simulink model "LabB_CheckCommunications"  (R2018b)
settings: Solver=FixedStepDiscrete  StartTime=0.0  StopTime=Inf  FixedStep=fSamplingPeriod  RelTol=1e-3  EnableMultiTasking=on
values from neighbouring files (symbols this model uses):
  fSamplingPeriod = 0.005    [LabB_ObserverOverSimulator_Discrete_Parameters.m]    (also in LabB_PIDOverRobot_Parameters.m)
undefined symbols (not defined in the file or in its folder): DiscIntNeverNeededParam
libraries: simulink_extras x3, MinSegLibrary_M2V3 x3
settings Model: SimulationMode=external  ExtModeTrigDuration=2  Creator=Alec  LastModifiedBy=pyry
settings DataIOCC: LimitDataPoints=on  SaveFormat=Array
settings OptimizationCC: PassReuseOutputArgsAs=Individual arguments  ExpressionDepthLimit=2147483647  MaxStackSize=64
settings DebuggingCC: UnderspecifiedInitializationDetection=Classic  MergeDetectMultiDrivingBlocksExec=none  ParameterTunabilityLossMsg=error  StateNameClashWarn=warning  SFUnexpectedBacktrackingDiag=warning  SFNoUnconditionalDefaultTransitionDiag=warning  SFExecutionAtInitializationDiag=none
settings HardwareCC: ProdBitPerInt=16  ProdBitPerPointer=16  ProdBitPerSizeT=16  ProdBitPerPtrDiffT=16  ProdLargestAtomicFloat=None  ProdWordSize=8  ProdHWDeviceType=Atmel->AVR
settings ModelReferenceCC: PropagateSignalLabelsOutOfModel=off
settings SFSimCC: SimUseLocalCustomCode=off  MATLABDynamicMemAlloc=off
settings RTWCC: SystemTargetFile=ert.tlc  HardwareBoard=Arduino Mega 2560  TemplateMakefile=ert_default_tmf  GenerateReport=on  RTWVerbose=off  RTWUseLocalCustomCode=off  Toolchain=Arduino AVR  BuildConfiguration=Faster Runs  IncludeHyperlinkInReport=on  LaunchReport=on  GenerateTraceInfo=on  GenerateTraceReport=on  GenerateTraceReportSl=on  GenerateTraceReportSf=on  GenerateTraceReportEml=on
settings CodeAppCC: ForceParamTrailComments=on  IgnoreCustomStorageClasses=off  OperatorAnnotations=on  SimulinkDataObjDesc=on  SFDataObjDesc=on  MATLABFcnDesc=on  CustomSymbolStrType=$N$R$M  InsertBlockDesc=on  StateflowObjectComments=on  MATLABSourceComments=on  InternalIdentifier=Classic
settings ERTTargetCC: SupportContinuousTime=on  SupportVariableSizeSignals=on
settings ConfigComp: CovMetricSettings=dw  CovHtmlReporting=on  CovSaveCumulativeToWorkspaceVar=on  CovSaveSingleToWorkspaceVar=on  CovExternalEMLEnable=off

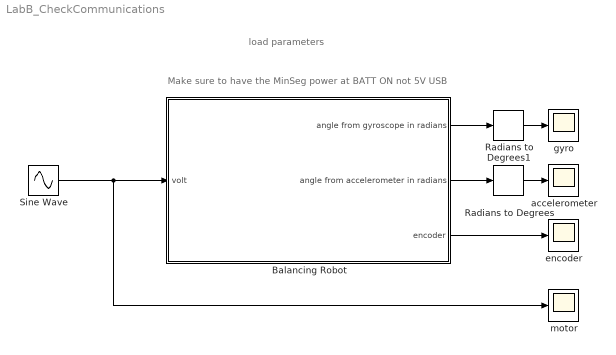
== system LabB_CheckCommunications ==
  note: Make sure to have the MinSeg power at BATT ON not 5V USB
  note: load parameters
  Balancing Robot : Subsystem
  Radians to Degrees : simulink_extras/Transformations/Radians to Degrees
  Radians to Degrees1 : simulink_extras/Transformations/Radians to Degrees
  Sine Wave : Sin  Amplitude=2  Frequency=pi/3  SampleTime=fSamplingPeriod
  accelerometer : Scope
  encoder : Scope
  gyro : Scope
  motor : Scope
  wires:
  Balancing Robot/1(angle from gyroscope in radians) -> Radians to Degrees1/1
  Balancing Robot/2(angle from accelerometer in radians) -> Radians to Degrees/1
  Balancing Robot/3(encoder) -> encoder/1
  Radians to Degrees1/1 -> gyro/1
  Radians to Degrees/1 -> accelerometer/1
  Sine Wave/1 -> motor/1, Balancing Robot/1(volt)

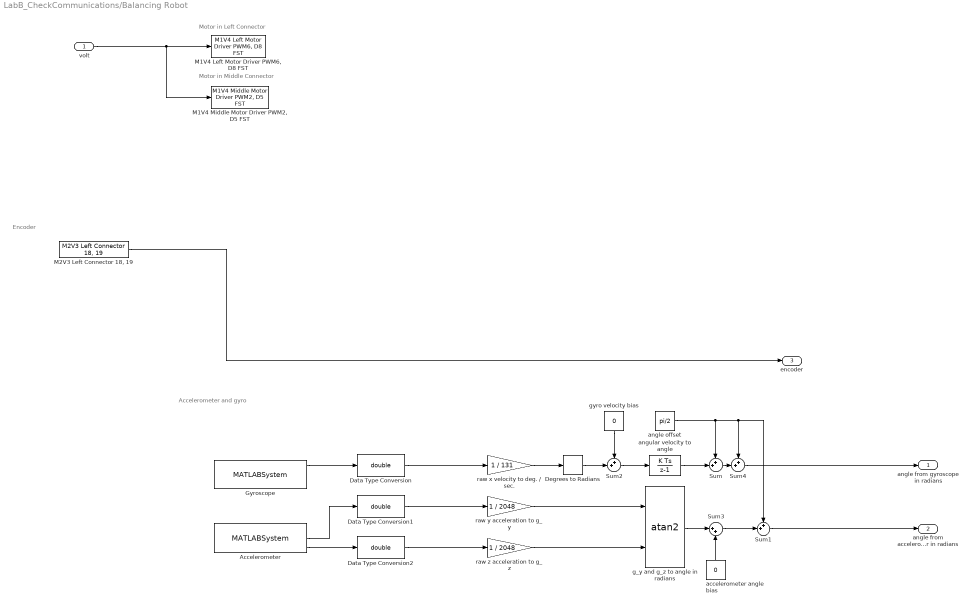
== system LabB_CheckCommunications/Balancing Robot ==
  note: Encoder
  note: Accelerometer and gyro
  note: Motor in Left Connector
  note: Motor in Middle Connector
  volt : Inport
  Accelerometer : MATLABSystem  System=soMPU6050Accel  SimulateUsing=Code generation
      mask Type: soMPU6050Accel
      mask Display:
      | disp('soMPU6050Accel');
      | port_label('output',1,'xaccel');
      | port_label('output',2,'yaccel');
      | port_label('output',3,'zaccel');
  Data Type Conversion : DataTypeConversion  OutDataTypeStr=double
  Data Type Conversion1 : DataTypeConversion  OutDataTypeStr=double
  Data Type Conversion2 : DataTypeConversion  OutDataTypeStr=double
  Degrees to Radians : simulink_extras/Transformations/Degrees to Radians
  Gyroscope : MATLABSystem  System=soMPU6050Gyro  DLPFmode=0
      mask Type: soMPU6050Gyro
      mask Display:
      | disp('soMPU6050Gyro');
      | port_label('output',1,'xvel');
      | port_label('output',2,'yvel');
      | port_label('output',3,'zvel');
  "M1V4 Left Motor Driver PWM6, D8 FST" : MinSegLibrary_M2V3/M1V4 Left Motor Driver PWM6, D8 FST  Vsupply=7.2
      settings: SourceProductName=Rensselaer Arduino Support Package
  "M1V4 Middle Motor Driver PWM2, D5 FST" : MinSegLibrary_M2V3/M1V4 Middle Motor Driver PWM2, D5 FST  Vsupply=7.2
      settings: SourceProductName=Rensselaer Arduino Support Package
  "M2V3 Left Connector 18, 19" : MinSegLibrary_M2V3/M2V3 Left Connector 18, 19  Encoder=1  PinA=19  PinB=18
      settings: SourceProductName=Rensselaer Arduino Support Package
  Sum{,1..2,4} (4 alike) : Sum  Inputs=++|
  Sum3 : Sum  Inputs=|++
  accelerometer angle bias : Constant  Value=0
  angle offset : Constant  Value=pi/2
  angular velocity to angle : DiscreteIntegrator  SampleTime=-1  ICPrevOutput=DiscIntNeverNeededParam  ICPrevScaledInput=DiscIntNeverNeededParam
  g_y and g_z to angle in radians : Trigonometry  Operator=atan2
  gyro velocity bias : Constant  Value=0
  raw x velocity to deg. / sec. : Gain  Gain=1 / 131
  raw y acceleration to g_y : Gain  Gain=1 / 2048
  raw z acceleration to g_z : Gain  Gain=1 / 2048
  angle from gyroscope in radians : Outport
  angle from accelerometer in radians : Outport  Port=2
  encoder : Outport  Port=3
  wires:
  Gyroscope/1 -> Data Type Conversion/1
  Accelerometer/2 -> Data Type Conversion1/1
  raw z acceleration to g_z/1 -> g_y and g_z to angle in radians/2
  raw y acceleration to g_y/1 -> g_y and g_z to angle in radians/1
  angle offset/1 -> Sum4/1, Sum1/1, Sum/1
  raw x velocity to deg. / sec./1 -> Degrees to Radians/1
  Sum/1 -> Sum4/2
  Data Type Conversion2/1 -> raw z acceleration to g_z/1
  Data Type Conversion1/1 -> raw y acceleration to g_y/1
  Data Type Conversion/1 -> raw x velocity to deg. / sec./1
  Accelerometer/3 -> Data Type Conversion2/1
  "M2V3 Left Connector 18, 19"/1 -> encoder/1
  Sum1/1 -> angle from accelerometer in radians/1
  angular velocity to angle/1 -> Sum/2
  Degrees to Radians/1 -> Sum2/2
  gyro velocity bias/1 -> Sum2/1
  Sum2/1 -> angular velocity to angle/1
  g_y and g_z to angle in radians/1 -> Sum3/1
  Sum3/1 -> Sum1/2
  accelerometer angle bias/1 -> Sum3/2
  Sum4/1 -> angle from gyroscope in radians/1
  volt/1 -> "M1V4 Middle Motor Driver PWM2, D5 FST"/1, "M1V4 Left Motor Driver PWM6, D8 FST"/1
